simulink model "classifyRealtimeTEST"  (R2019a)
settings: Solver=VariableStepAuto  StartTime=0.0  StopTime=inf  RelTol=1e-3
undefined symbols (not defined in the file or in its folder): daq
libraries: daqlib x1, dspxfrm3 x1, dspnetwork x1
settings Model: Creator=Kusunoki  LastModifiedBy=Owner

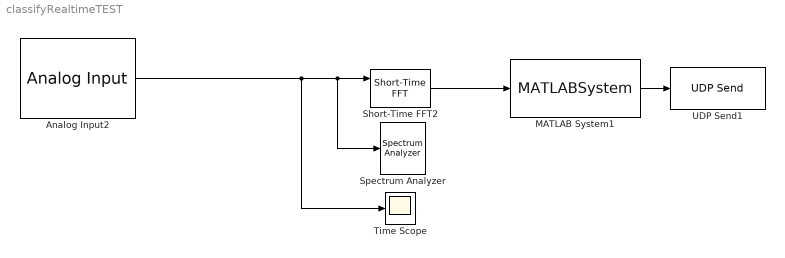
== system classifyRealtimeTEST ==
  Analog Input2 : daqlib/Analog Input  DeviceMenu=ni Dev1 (USB-6000)  Device=ni Dev1 (USB-6000)  ObjConstructor=daq.createSession('ni')  NChannelsSelected=1  Channels=1$ai0$$Dev1$1$1$1$1$#0$ai1$$Dev1$1$1$1$1$#0$ai2$$Dev1$1$1$1$1$#0$ai3$$Dev1$1$1$1$1$#0$ai4$$Dev1$1$1$1$1$#0$ai5$$Dev1$1$1$1$1$#0$ai6$$Dev1$1$1$1$1$#0$ai7$$Dev1$1$1$1$1$#  NPorts=1 per channel  SampleRate=2000  ActualRate=2000  ScansPerTrigger=200  OutputTimestamp=off  AcqMode=0  NumFrameBuffer=100  OutputTriggertime=off
      settings: SourceProductName=Data Acquisition Toolbox  SourceProductBaseCode=DA
  MATLAB System1 : MATLABSystem  System=NetTEST  net=[]  SimulateUsing=Code generation
      mask Type: NetTEST
      mask Display:
      | disp('NetTEST');
      | port_label('input',1,'u');
      | port_label('output',1,'y');
  Short-Time FFT2 : dspxfrm3/Short-Time FFT  W=512  OvLap=384  M=1024
      settings: SourceProductName=DSP System Toolbox  SourceProductBaseCode=DS
  Spectrum Analyzer : SpectrumAnalyzer
  Time Scope : Scope
  UDP Send1 : dspnetwork/UDP Send  remoteURL='127.0.0.1'  remotePort=25000  localURL='0.0.0.0'  localPortSource=Automatically determine  localPort=-1  sampletime=-1  blockPlatform=[]  separateLengthPort=0
      settings: SourceProductName=Simulink
  wires:
  Analog Input2/1 -> Time Scope/1, Spectrum Analyzer/1, Short-Time FFT2/1
  MATLAB System1/1 -> UDP Send1/1
  Short-Time FFT2/1 -> MATLAB System1/1
